simulink model "CnvSet_Trq2Q"  (R2016b)
settings: configuration reference "CodeGenConfigSet" (kept outside this file)
values from neighbouring files (symbols this model uses):
  CnvSet_eta0_C = Calibration.Parameter    [init_CnvSet_Trq2Q.m]    (also in init_CnvSet_Trq2Q_SIL.m = Simulink.Parameter)
  CnvSet_etaMax_C = Calibration.Parameter    [init_CnvSet_Trq2Q.m]    (also in init_CnvSet_Trq2Q_SIL.m = Simulink.Parameter)
  CnvSet_etaMin_C = Calibration.Parameter    [init_CnvSet_Trq2Q.m]    (also in init_CnvSet_Trq2Q_SIL.m = Simulink.Parameter)
  CnvSet_facRmpVal_CUR = Calibration.Parameter    [init_CnvSet_Trq2Q.m]    (also in init_CnvSet_Trq2Q_SIL.m = Simulink.Parameter)
  CnvSet_facRmpVal_CURX = Calibration.Parameter    [init_CnvSet_Trq2Q.m]    (also in init_CnvSet_Trq2Q_SIL.m = Simulink.Parameter)
  INJ_MASS_ZERO = fi(0,FuelMass_mg_hub)    [init_CnvSet_Trq2Q.m]    (also in init_CnvSet_Trq2Q_SIL.m)
  PhyMod_trq2qBas_MAP = Calibration.Parameter    [init_CnvSet_Trq2Q.m]    (also in init_CnvSet_Trq2Q_SIL.m = Simulink.Parameter)
  PhyMod_trq2qBas_MAPX = Calibration.Parameter    [init_CnvSet_Trq2Q.m]    (also in init_CnvSet_Trq2Q_SIL.m = Simulink.Parameter)
  PhyMod_trq2qBas_MAPY = Calibration.Parameter    [init_CnvSet_Trq2Q.m]    (also in init_CnvSet_Trq2Q_SIL.m = Simulink.Parameter)
libraries: CXLib x4, simulink x2
settings Model: Creator=Colin  LastModifiedBy=xuxingpei
settings ConfigSetRef: SourceLocation=Base Workspace

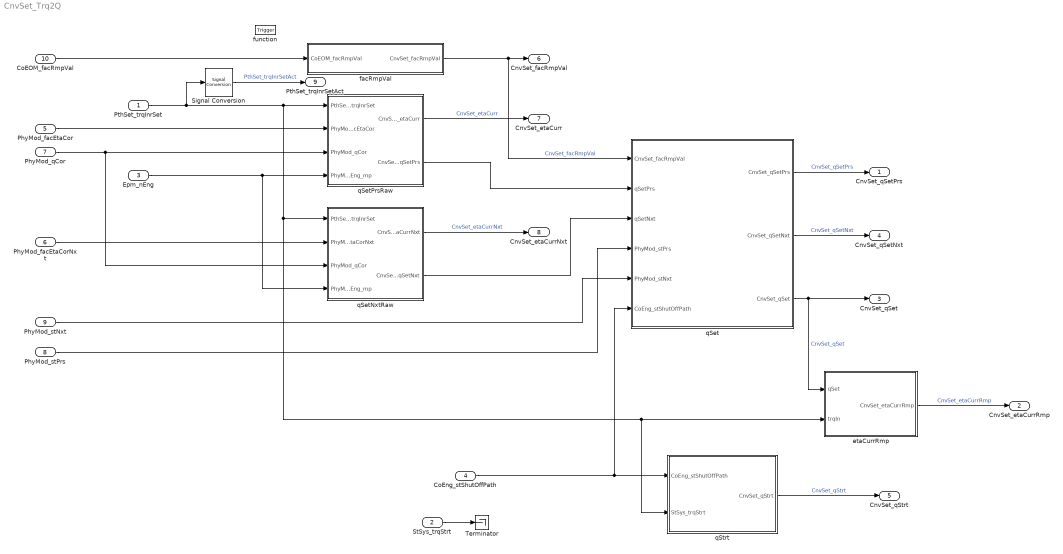
== system CnvSet_Trq2Q ==
  PthSet_trqInrSet : Inport  Tag=Nm  Description=Inner torque set value after monitoring limitation  OutMin=-3000  OutMax=3276.7  OutDataTypeStr=Trq_Nm
  StSys_trqStrt : Inport  Tag=Nm  Description=Engine starting torque  Port=2  OutMin=-3000  OutMax=3000  OutDataTypeStr=Trq_Nm
  Epm_nEng : Inport  Tag=rpm  Description=Engine speed  Port=3  OutMin=0  OutMax=6000  OutDataTypeStr=EngSpeed_rpm
  CoEng_stShutOffPath : Inport  Description=Active shut-off paths resulting from active reversible,irreversible and afterrun shut-off paths  Port=4  OutMin=0  OutMax=65535  OutDataTypeStr=State_uint16
  PhyMod_facEtaCor : Inport  Description=Current efficiency correction factor  Port=5  OutMin=-30  OutMax=30  OutDataTypeStr=Factor
  PhyMod_facEtaCorNxt : Inport  Description=next efficiency correction factor  Port=6  OutMin=-31  OutMax=31  OutDataTypeStr=Factor
  PhyMod_qCor : Inport  Tag=mg/hub  Description=Correction quantity  Port=7  OutMin=-319  OutMax=319  OutDataTypeStr=FuelMass_mg_hub
  PhyMod_stPrs : Inport  Description=Current operating mode for the torque structure  Port=8  OutMin=0  OutMax=255  OutDataTypeStr=State_uint8
  PhyMod_stNxt : Inport  Description=Next operating mode for the torque structure  Port=9  OutMin=0  OutMax=255  OutDataTypeStr=State_uint8
  CoEOM_facRmpVal : Inport  Description=Central ramp value for operation mode change  Port=10  OutMin=-31  OutMax=31  OutDataTypeStr=Factor
  function : TriggerPort  TriggerType=function-call  VariantControl=Variant
  Signal Conversion : SignalConversion  OverrideOpt=off
  Terminator : Terminator
  etaCurrRmp : Subsystem
  facRmpVal : Subsystem
  qSet : Subsystem
  qSetNxtRaw : Subsystem
  qSetPrsRaw : Subsystem
  qStrt : Subsystem
  CnvSet_qSetPrs : Outport  Tag=mg/hub  Description=Setpoint injection quantity current operation mode  OutMin=-319  OutMax=319  OutDataTypeStr=FuelMass_mg_hub
  CnvSet_etaCurrRmp : Outport  Tag=Nm/(mg/hub)  Description=Conversion efficiency corresponding to CnvSet_qSet  Port=2  OutMin=-255  OutMax=255  OutDataTypeStr=TrqEta_Nm_mg_hub
  CnvSet_qSet : Outport  Tag=mg/hub  Description=Set point injection quantity  Port=3  OutMin=-319  OutMax=319  OutDataTypeStr=FuelMass_mg_hub
  CnvSet_qSetNxt : Outport  Tag=mg/hub  Description=Setpoint injection quantity next opration mode  Port=4  OutMin=-319  OutMax=319  OutDataTypeStr=FuelMass_mg_hub
  CnvSet_qStrt : Outport  Tag=mg/hub  Description=Injection start quantity  Port=5  OutMin=-319  OutMax=319  OutDataTypeStr=FuelMass_mg_hub
  CnvSet_facRmpVal : Outport  Description=ramp value for operation mode switchover  Port=6  OutMin=-31  OutMax=31  OutDataTypeStr=Factor
  CnvSet_etaCurr : Outport  Tag=Nm/(mg/hub)  Description=Current conversion efficiency  Port=7  OutMin=-255  OutMax=255  OutDataTypeStr=TrqEta_Nm_mg_hub
  CnvSet_etaCurrNxt : Outport  Tag=Nm/(mg/hub)  Description=conversion efficiency for next operation mode  Port=8  OutMin=-255  OutMax=255  OutDataTypeStr=TrqEta_Nm_mg_hub
  PthSet_trqInrSetAct : Outport  Tag=Nm  Description=Current inner engine torque  Port=9  OutMin=-3276.8  OutMax=3276.7  OutDataTypeStr=Trq_Nm
  wires:
  facRmpVal/1(CnvSet_facRmpVal) -> CnvSet_facRmpVal/1, qSet/1(CnvSet_facRmpVal)  "CnvSet_facRmpVal"
  CoEOM_facRmpVal/1 -> facRmpVal/1(CoEOM_facRmpVal)
  PhyMod_facEtaCor/1 -> qSetPrsRaw/2(PhyMod_facEtaCor)
  Epm_nEng/1 -> qSetNxtRaw/4(PhyMod_nEng_mp), qSetPrsRaw/4(PhyMod_nEng_mp)
  qSetPrsRaw/1(CnvSet_etaCurr) -> CnvSet_etaCurr/1  "CnvSet_etaCurr"
  PhyMod_facEtaCorNxt/1 -> qSetNxtRaw/2(PhyMod_facEtaCorNxt)
  PhyMod_qCor/1 -> qSetNxtRaw/3(PhyMod_qCor), qSetPrsRaw/3(PhyMod_qCor)
  qSetNxtRaw/1(CnvSet_etaCurrNxt) -> CnvSet_etaCurrNxt/1  "CnvSet_etaCurrNxt"
  qStrt/1(CnvSet_qStrt) -> CnvSet_qStrt/1  "CnvSet_qStrt"
  etaCurrRmp/1(CnvSet_etaCurrRmp) -> CnvSet_etaCurrRmp/1  "CnvSet_etaCurrRmp"
  qSet/1(CnvSet_qSetPrs) -> CnvSet_qSetPrs/1  "CnvSet_qSetPrs"
  qSet/3(CnvSet_qSet) -> etaCurrRmp/1(qSet), CnvSet_qSet/1  "CnvSet_qSet"
  qSet/2(CnvSet_qSetNxt) -> CnvSet_qSetNxt/1  "CnvSet_qSetNxt"
  PhyMod_stNxt/1 -> qSet/5(PhyMod_stNxt)
  PhyMod_stPrs/1 -> qSet/4(PhyMod_stPrs)
  qSetNxtRaw/2(CnvSet_qSetNxt) -> qSet/3(qSetNxt)
  qSetPrsRaw/2(CnvSet_qSetPrs) -> qSet/2(qSetPrs)
  CoEng_stShutOffPath/1 -> qStrt/1(CoEng_stShutOffPath), qSet/6(CoEng_stShutOffPath)
  PthSet_trqInrSet/1 -> Signal Conversion/1, qStrt/2(StSys_trqStrt), etaCurrRmp/2(trqIn), qSetNxtRaw/1(PthSet_trqInrSet), qSetPrsRaw/1(PthSet_trqInrSet)
  Signal Conversion/1 -> PthSet_trqInrSetAct/1  "PthSet_trqInrSetAct"
  StSys_trqStrt/1 -> Terminator/1

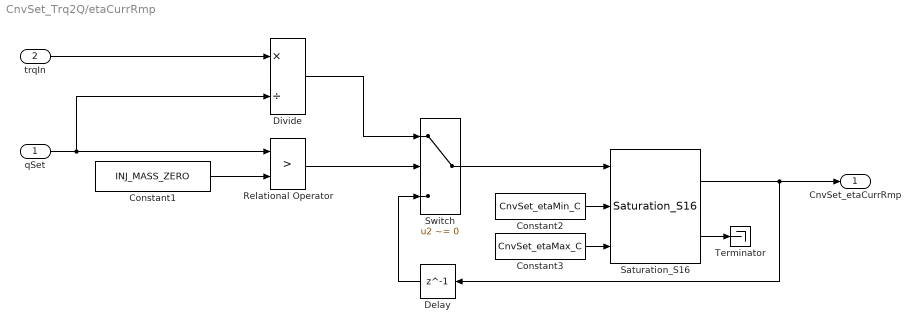
== system CnvSet_Trq2Q/etaCurrRmp ==
  qSet : Inport
  trqIn : Inport  Port=2
  Constant1 : Constant  Value=INJ_MASS_ZERO
  Constant2 : Constant  Value=CnvSet_etaMin_C
  Constant3 : Constant  Value=CnvSet_etaMax_C
  Delay : Delay  DelayLength=1  InitialCondition=0
  Divide : Product  Inputs=*/  OutDataTypeStr=TrqEta_Nm_mg_hub  SaturateOnIntegerOverflow=on
  Relational Operator : RelationalOperator  Operator=>  OutDataTypeStr=boolean  RndMeth=Simplest
  Saturation_S16 : CXLib/Saturation_S16
  Switch : Switch  Criteria=u2 ~= 0  OutDataTypeStr=Inherit: Inherit via back propagation  InputSameDT=on
  Terminator : Terminator
  CnvSet_etaCurrRmp : Outport
  wires:
  qSet/1 -> Divide/2, Relational Operator/1
  Constant1/1 -> Relational Operator/2
  trqIn/1 -> Divide/1
  Relational Operator/1 -> Switch/2
  Divide/1 -> Switch/1
  Delay/1 -> Switch/3
  Saturation_S16/2 -> Terminator/1
  Constant2/1 -> Saturation_S16/2
  Constant3/1 -> Saturation_S16/3
  Saturation_S16/1 -> Delay/1, CnvSet_etaCurrRmp/1
  Switch/1 -> Saturation_S16/1

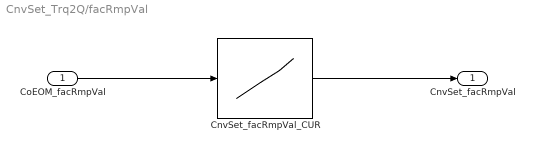
== system CnvSet_Trq2Q/facRmpVal ==
  CoEOM_facRmpVal : Inport
  CnvSet_facRmpVal_CUR : Lookup_n-D  NumberOfTableDimensions=1  BreakpointsForDimension1=CnvSet_facRmpVal_CURX  Table=CnvSet_facRmpVal_CUR  ExtrapMethod=Clip  InternalRulePriority=Speed  OutDataTypeStr=Inherit: Inherit via back propagation  RndMeth=Simplest  InputSameDT=on
  CnvSet_facRmpVal : Outport
  wires:
  CoEOM_facRmpVal/1 -> CnvSet_facRmpVal_CUR/1
  CnvSet_facRmpVal_CUR/1 -> CnvSet_facRmpVal/1

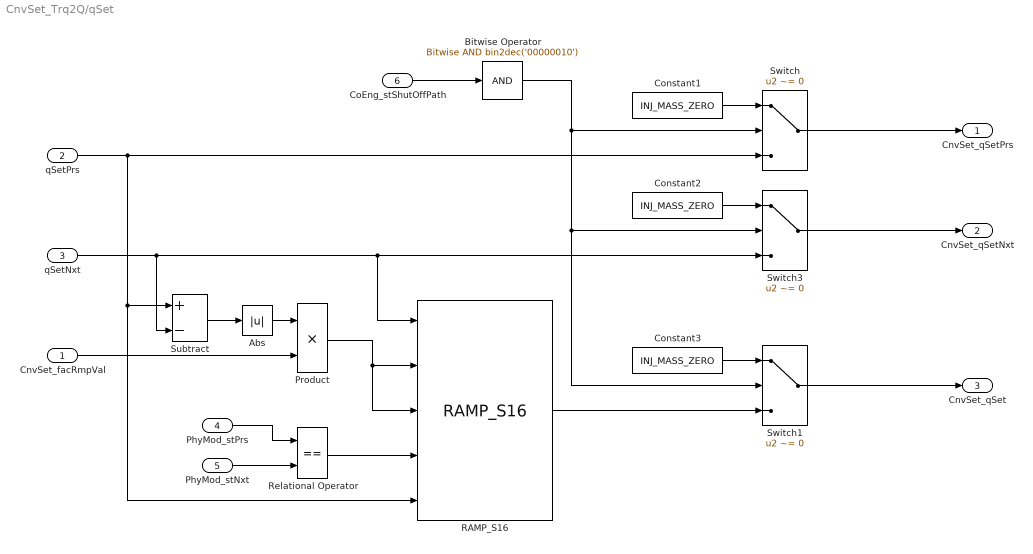
== system CnvSet_Trq2Q/qSet ==
  CnvSet_facRmpVal : Inport
  qSetPrs : Inport  Port=2
  qSetNxt : Inport  Port=3
  PhyMod_stPrs : Inport  Port=4
  PhyMod_stNxt : Inport  Port=5
  CoEng_stShutOffPath : Inport  Port=6
  Abs : Abs
  Bitwise Operator : simulink/Logic and Bit Operations/Bitwise Operator  logicop=AND  UseBitMask=on  BitMask=bin2dec('00000010')  BitMaskRealWorld=Stored Integer
  Constant1 : Constant  Value=INJ_MASS_ZERO  OutDataTypeStr=Inherit: Inherit via back propagation
  Constant2 : Constant  Value=INJ_MASS_ZERO  OutDataTypeStr=Inherit: Inherit via back propagation
  Constant3 : Constant  Value=INJ_MASS_ZERO  OutDataTypeStr=Inherit: Inherit via back propagation
  Product : Product  OutDataTypeStr=FuelMass_mg_hub  SaturateOnIntegerOverflow=on
  RAMP_S16 : CXLib/RAMP_S16
  Relational Operator : RelationalOperator  Operator===  OutDataTypeStr=boolean  RndMeth=Simplest
  Subtract : Sum  Inputs=+-  SaturateOnIntegerOverflow=on
  Switch : Switch  Criteria=u2 ~= 0  OutDataTypeStr=Inherit: Inherit via back propagation
  Switch1 : Switch  Criteria=u2 ~= 0  OutDataTypeStr=Inherit: Inherit via back propagation
  Switch3 : Switch  Criteria=u2 ~= 0  OutDataTypeStr=Inherit: Inherit via back propagation
  CnvSet_qSetPrs : Outport
  CnvSet_qSetNxt : Outport  Port=2
  CnvSet_qSet : Outport  Port=3
  wires:
  CoEng_stShutOffPath/1 -> Bitwise Operator/1
  Switch/1 -> CnvSet_qSetPrs/1
  Bitwise Operator/1 -> Switch1/2, Switch3/2, Switch/2
  Constant1/1 -> Switch/1
  qSetPrs/1 -> RAMP_S16/5, Subtract/1, Switch/3
  Switch3/1 -> CnvSet_qSetNxt/1
  qSetNxt/1 -> Subtract/2, RAMP_S16/1, Switch3/3
  Constant2/1 -> Switch3/1
  PhyMod_stPrs/1 -> Relational Operator/1
  PhyMod_stNxt/1 -> Relational Operator/2
  Relational Operator/1 -> RAMP_S16/4
  Subtract/1 -> Abs/1
  Abs/1 -> Product/1
  CnvSet_facRmpVal/1 -> Product/2
  Product/1 -> RAMP_S16/3, RAMP_S16/2
  RAMP_S16/1 -> Switch1/3
  Constant3/1 -> Switch1/1
  Switch1/1 -> CnvSet_qSet/1

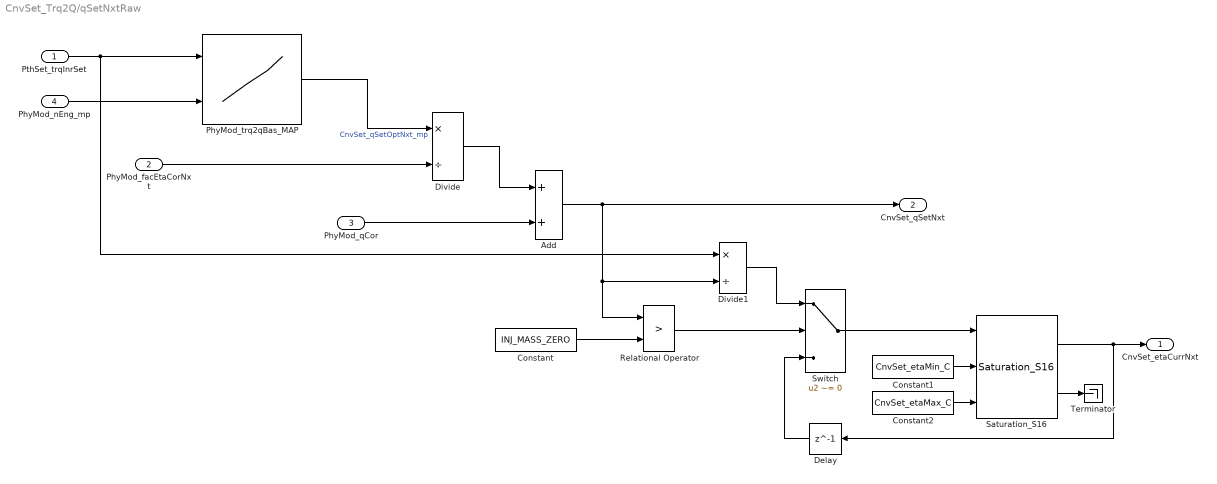
== system CnvSet_Trq2Q/qSetNxtRaw ==
  PthSet_trqInrSet : Inport
  PhyMod_facEtaCorNxt : Inport  Port=2
  PhyMod_qCor : Inport  Port=3
  PhyMod_nEng_mp : Inport  Port=4
  Add : Sum  OutDataTypeStr=FuelMass_mg_hub  SaturateOnIntegerOverflow=on  InputSameDT=on
  Constant : Constant  Value=INJ_MASS_ZERO
  Constant1 : Constant  Value=CnvSet_etaMin_C
  Constant2 : Constant  Value=CnvSet_etaMax_C
  Delay : Delay  DelayLength=1  InitialCondition=0
  Divide : Product  Inputs=*/  OutDataTypeStr=FuelMass_mg_hub  SaturateOnIntegerOverflow=on
  Divide1 : Product  Inputs=*/  OutDataTypeStr=TrqEta_Nm_mg_hub  SaturateOnIntegerOverflow=on
  PhyMod_trq2qBas_MAP : Lookup_n-D  BreakpointsForDimension1=PhyMod_trq2qBas_MAPY  BreakpointsForDimension2=PhyMod_trq2qBas_MAPX  Table=PhyMod_trq2qBas_MAP  ExtrapMethod=Clip  InternalRulePriority=Speed  OutDataTypeStr=FuelMass_mg_hub  RndMeth=Simplest
  Relational Operator : RelationalOperator  Operator=>  OutDataTypeStr=boolean  RndMeth=Simplest
  Saturation_S16 : CXLib/Saturation_S16
  Switch : Switch  Criteria=u2 ~= 0  OutDataTypeStr=Inherit: Inherit via back propagation  InputSameDT=on
  Terminator : Terminator
  CnvSet_etaCurrNxt : Outport
  CnvSet_qSetNxt : Outport  Port=2
  wires:
  PhyMod_trq2qBas_MAP/1 -> Divide/1  "CnvSet_qSetOptNxt_mp"
  PhyMod_facEtaCorNxt/1 -> Divide/2
  Divide/1 -> Add/1
  PhyMod_qCor/1 -> Add/2
  Constant/1 -> Relational Operator/2
  Relational Operator/1 -> Switch/2
  Divide1/1 -> Switch/1
  Add/1 -> CnvSet_qSetNxt/1, Divide1/2, Relational Operator/1
  PthSet_trqInrSet/1 -> Divide1/1, PhyMod_trq2qBas_MAP/1
  PhyMod_nEng_mp/1 -> PhyMod_trq2qBas_MAP/2
  Delay/1 -> Switch/3
  Saturation_S16/2 -> Terminator/1
  Constant1/1 -> Saturation_S16/2
  Constant2/1 -> Saturation_S16/3
  Saturation_S16/1 -> Delay/1, CnvSet_etaCurrNxt/1
  Switch/1 -> Saturation_S16/1

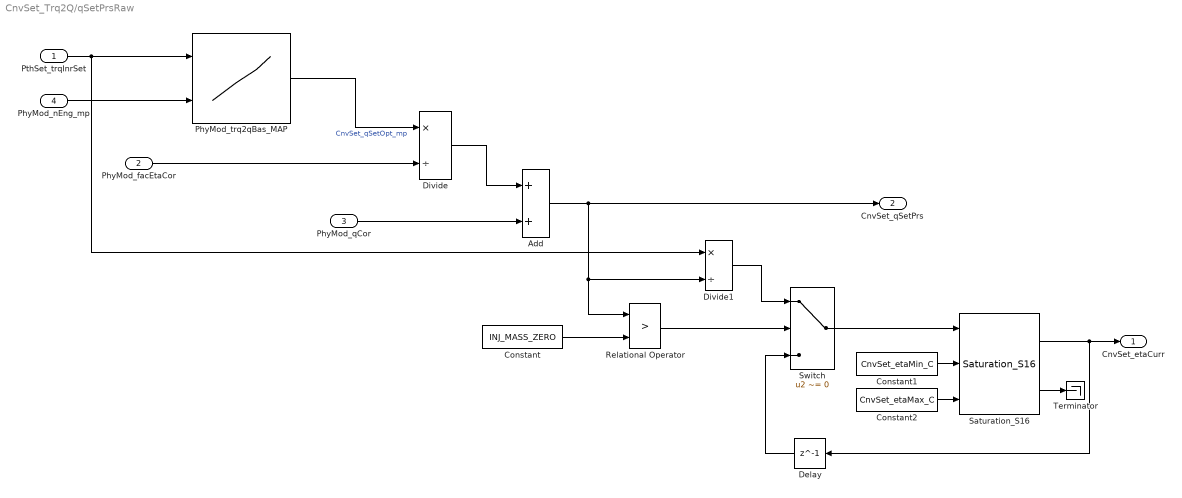
== system CnvSet_Trq2Q/qSetPrsRaw ==
  PthSet_trqInrSet : Inport
  PhyMod_facEtaCor : Inport  Port=2
  PhyMod_qCor : Inport  Port=3
  PhyMod_nEng_mp : Inport  Port=4
  Add : Sum  OutDataTypeStr=FuelMass_mg_hub  SaturateOnIntegerOverflow=on  InputSameDT=on
  Constant : Constant  Value=INJ_MASS_ZERO
  Constant1 : Constant  Value=CnvSet_etaMin_C
  Constant2 : Constant  Value=CnvSet_etaMax_C
  Delay : Delay  DelayLength=1  InitialCondition=0
  Divide : Product  Inputs=*/  OutDataTypeStr=FuelMass_mg_hub  SaturateOnIntegerOverflow=on
  Divide1 : Product  Inputs=*/  OutDataTypeStr=TrqEta_Nm_mg_hub  SaturateOnIntegerOverflow=on
  PhyMod_trq2qBas_MAP : Lookup_n-D  BreakpointsForDimension1=PhyMod_trq2qBas_MAPY  BreakpointsForDimension2=PhyMod_trq2qBas_MAPX  Table=PhyMod_trq2qBas_MAP  ExtrapMethod=Clip  InternalRulePriority=Speed  OutDataTypeStr=FuelMass_mg_hub  RndMeth=Simplest
  Relational Operator : RelationalOperator  Operator=>  OutDataTypeStr=boolean  RndMeth=Simplest
  Saturation_S16 : CXLib/Saturation_S16
  Switch : Switch  Criteria=u2 ~= 0  OutDataTypeStr=Inherit: Inherit via back propagation  InputSameDT=on
  Terminator : Terminator
  CnvSet_etaCurr : Outport
  CnvSet_qSetPrs : Outport  Port=2
  wires:
  PthSet_trqInrSet/1 -> Divide1/1, PhyMod_trq2qBas_MAP/1
  PhyMod_trq2qBas_MAP/1 -> Divide/1  "CnvSet_qSetOpt_mp"
  PhyMod_facEtaCor/1 -> Divide/2
  Divide/1 -> Add/1
  PhyMod_qCor/1 -> Add/2
  Constant/1 -> Relational Operator/2
  Relational Operator/1 -> Switch/2
  Divide1/1 -> Switch/1
  Add/1 -> Divide1/2, Relational Operator/1, CnvSet_qSetPrs/1
  PhyMod_nEng_mp/1 -> PhyMod_trq2qBas_MAP/2
  Delay/1 -> Switch/3
  Switch/1 -> Saturation_S16/1
  Saturation_S16/1 -> Delay/1, CnvSet_etaCurr/1
  Saturation_S16/2 -> Terminator/1
  Constant1/1 -> Saturation_S16/2
  Constant2/1 -> Saturation_S16/3

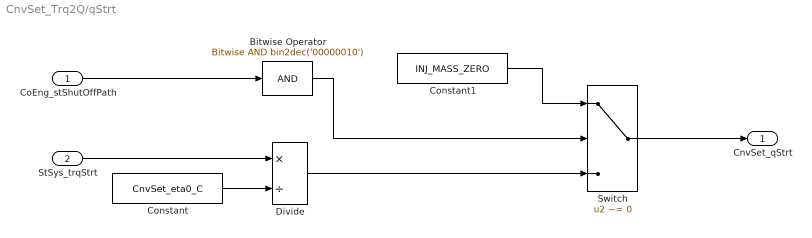
== system CnvSet_Trq2Q/qStrt ==
  CoEng_stShutOffPath : Inport
  StSys_trqStrt : Inport  Port=2
  Bitwise Operator : simulink/Logic and Bit Operations/Bitwise Operator  logicop=AND  UseBitMask=on  BitMask=bin2dec('00000010')  BitMaskRealWorld=Stored Integer
  Constant : Constant  Value=CnvSet_eta0_C
  Constant1 : Constant  Value=INJ_MASS_ZERO
  Divide : Product  Inputs=*/  OutDataTypeStr=Inherit: Inherit via back propagation  SaturateOnIntegerOverflow=on
  Switch : Switch  Criteria=u2 ~= 0  OutDataTypeStr=Inherit: Inherit via back propagation
  CnvSet_qStrt : Outport
  wires:
  Switch/1 -> CnvSet_qStrt/1
  Constant1/1 -> Switch/1
  StSys_trqStrt/1 -> Divide/1
  Constant/1 -> Divide/2
  Divide/1 -> Switch/3
  CoEng_stShutOffPath/1 -> Bitwise Operator/1
  Bitwise Operator/1 -> Switch/2
